simulink model "sistemaMotorCC_RNA"  (R2018a)
settings: Solver=FixedStepAuto  StartTime=0.0  StopTime=119.98  RelTol=1e-3
PreLoadFcn:
  | % Motor Parameters
  | 
  | J=0.01;     %kg*m^2
  | b=0.1;      %N*m/(rad/s)
  | K=0.01;     %V/(rad/s)
  | R=1;        %Ohm
  | L=0.5;      %H
settings Model: Creator=deastman  LastModifiedBy=artur
settings DataIOCC: LimitDataPoints=on  SaveFormat=Array
settings OptimizationCC: ExpressionDepthLimit=2147483647  InitFltsAndDblsToZero=on  LifeSpan=inf
settings DebuggingCC: UnderspecifiedInitializationDetection=Classic  MergeDetectMultiDrivingBlocksExec=none  SolverPrmCheckMsg=warning  FcnCallInpInsideContextMsg=warning  StateNameClashWarn=warning  SFUnexpectedBacktrackingDiag=warning  SFNoUnconditionalDefaultTransitionDiag=warning  SFExecutionAtInitializationDiag=none
settings HardwareCC: ProdBitPerPointer=32  ProdBitPerSizeT=32  ProdBitPerPtrDiffT=32  ProdLargestAtomicFloat=None  ProdIntDivRoundTo=Undefined  ProdEndianess=Unspecified  ProdWordSize=32  ProdHWDeviceType=32-bit Generic
settings ModelReferenceCC: PropagateSignalLabelsOutOfModel=off
settings CodeAppCC: StateflowObjectComments=on
settings GRTTargetCC: TargetLangStandard=C89/C90 (ANSI)  GeneratePreprocessorConditionals=Disable all  CombineOutputUpdateFcns=off  GRTInterface=on
settings ConfigComp: CovMetricSettings=dw  CovHtmlReporting=on  CovSaveCumulativeToWorkspaceVar=on  CovSaveSingleToWorkspaceVar=on  CovExternalEMLEnable=off

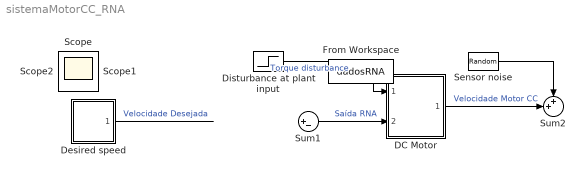
== system sistemaMotorCC_RNA ==
  " Disturbance at plant input" : Step  Time=0  After=0  SampleTime=0
  DC Motor : Subsystem  mask(DC Motor){b=b, J=J, K=K, R=R, L=L}
      mask prompts: b "Damping:"; J "Inertia:"; K "Back EMF:"; R "Resistance:"; L "Inductance:"
      mask help: An ideal model of a DC Motor
      mask Help: This is <b>more elaborate<b> help.
      mask Display: image(imread('dcmotor.jpg'))
  Desired speed : Subsystem
  Sensor noise : RandomNumber  Variance=0  SampleTime=0
  Sum1 : Sum  Inputs=|+-
  Sum2 : Sum  Inputs=++|
  From Workspace : FromWorkspace  IOType=siggen  VariableName=dadosRNA  SampleTime=0.02  Interpolate=off  OutputAfterFinalValue=Holding final value
  Scope : Scope
  Scope1 : Scope
  Scope2 : Scope
  wires:
  " Disturbance at plant input"/1 -> DC Motor/1(Torque)  "Torque disturbance"
  Desired speed/1(Speed) -> ?  "Velocidade Desejada"
  DC Motor/1(Speed) -> Sum2/2  "Velocidade Motor CC"
  Sensor noise/1 -> Sum2/1
  Sum1/1 -> DC Motor/2(Voltage)  "Saída RNA"

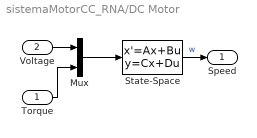
== system sistemaMotorCC_RNA/DC Motor ==
  Torque : Inport
  Voltage : Inport  Port=2
  Mux : Mux  Inputs=2
  State-Space : StateSpace  A=[-b/J K/J; -K/L -R/L]  B=[0 -1/J; 1/L 0]  C=[1 0]  D=[0 0]  InitialCondition=0
  Speed : Outport
  wires:
  Mux/1 -> State-Space/1
  Voltage/1 -> Mux/1
  State-Space/1 -> Speed/1  "w"
  Torque/1 -> Mux/2

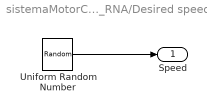
== system sistemaMotorCC_RNA/Desired speed ==
  Uniform Random Number : UniformRandomNumber  Minimum=-5  Maximum=5  Seed=1  SampleTime=6
  Speed : Outport
  wires:
  Uniform Random Number/1 -> Speed/1
